simulink model "dc"  (Simulink 7.0)
settings: Solver=ode45  StartTime=0.0  StopTime=3.0  RelTol=1e-3
settings Model: Creator=User  LastModifiedBy=azad

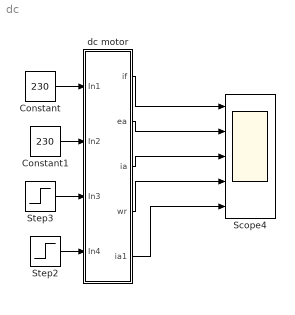
== system dc ==
  Constant : Constant  Value=230  OutDataType=sfix(16)  OutScaling=2^0
  Constant1 : Constant  Value=230  OutDataType=sfix(16)  OutScaling=2^0
  Scope4 : Scope  NumInputPorts=5
      settings: YMin=0~0~0~0~-5  YMax=1~30~400~17.5~5  SaveName=ScopeData4
  Step2 : Step  Time=1.5  After=-250  SampleTime=0
  Step3 : Step  After=250  SampleTime=0
  dc motor : Subsystem  mask{ra=0.6, rf=240, la=0.012, lf=120, laf=1.8, b=1.5, j=0.1}
      mask prompts: ra "ra(ohm)"; rf "rf(ohm)"; la "la(H)"; lf "lf(H)"; laf "laf(H)"; b "b(N.m.s)"; j "j(kg.m^2)"
  wires:
  Constant/1 -> dc motor/1(In1)
  Constant1/1 -> dc motor/2(In2)
  Step3/1 -> dc motor/3(In3)
  Step2/1 -> dc motor/4(In4)
  dc motor/1(if) -> Scope4/1
  dc motor/2(ea) -> Scope4/2
  dc motor/3(ia) -> Scope4/3
  dc motor/4(wr) -> Scope4/4
  dc motor/5(ia1) -> Scope4/5

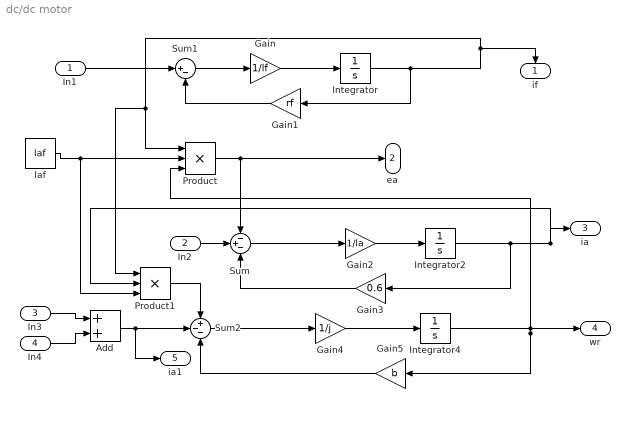
== system dc/dc motor ==
  In1 : Inport
  In2 : Inport  Port=2
  In3 : Inport  Port=3
  In4 : Inport  Port=4
  Add : Sum  OutDataType=sfix(16)  OutScaling=2^-10
  Gain : Gain  Gain=1/lf  ParameterDataType=sfix(16)  ParameterScaling=2^0  OutDataType=sfix(16)  OutScaling=2^0
  Gain1 : Gain  Orientation=left  Gain=rf  ParameterDataType=sfix(16)  ParameterScaling=2^0  OutDataType=sfix(16)  OutScaling=2^0
  Gain2 : Gain  Gain=1/la  ParameterDataType=sfix(16)  ParameterScaling=2^0  OutDataType=sfix(16)  OutScaling=2^0
  Gain3 : Gain  Orientation=left  Gain=0.6  ParameterDataType=sfix(16)  ParameterScaling=2^0  OutDataType=sfix(16)  OutScaling=2^0
  Gain4 : Gain  Gain=1/j  ParameterDataType=sfix(16)  ParameterScaling=2^0  OutDataType=sfix(16)  OutScaling=2^0
  Gain5 : Gain  Orientation=left  Gain=b  ParameterDataType=sfix(16)  ParameterScaling=2^0  OutDataType=sfix(16)  OutScaling=2^0
  Integrator : Integrator
  Integrator2 : Integrator
  Integrator4 : Integrator
  Product : Product  Inputs=3  OutDataType=sfix(16)  OutScaling=2^0  RndMeth=Zero
  Product1 : Product  Inputs=3  OutDataType=sfix(16)  OutScaling=2^0  RndMeth=Zero
  Sum : Sum  Inputs=-+-  OutDataType=sfix(16)  OutScaling=2^0
  Sum1 : Sum  Inputs=|+-  OutDataType=sfix(16)  OutScaling=2^0
  Sum2 : Sum  Inputs=+--  OutDataType=sfix(16)  OutScaling=2^0
  laf : Constant  Value=laf  OutDataType=sfix(16)  OutScaling=2^0
  if : Outport  Orientation=down
  ea : Outport  Port=2
  ia : Outport  Port=3
  wr : Outport  Port=4
  ia1 : Outport  Port=5  OutDataType=sfix(16)  OutScaling=2^0
  wires:
  Gain/1 -> Integrator/1
  Integrator/1 -> Product/1, Product1/1, if/1, Gain1/1
  Sum1/1 -> Gain/1
  Gain1/1 -> Sum1/2
  Gain2/1 -> Integrator2/1
  Sum/1 -> Gain2/1
  Integrator2/1 -> Gain3/1, Product1/2, ia/1
  Gain3/1 -> Sum/3
  Product/1 -> Sum/1, ea/1
  laf/1 -> Product/2, Product1/3
  Sum2/1 -> Gain4/1
  Gain4/1 -> Integrator4/1
  Gain5/1 -> Sum2/3
  Add/1 -> Sum2/2, ia1/1
  Product1/1 -> Sum2/1
  Integrator4/1 -> Product/3, wr/1, Gain5/1
  In1/1 -> Sum1/1
  In2/1 -> Sum/2
  In3/1 -> Add/1
  In4/1 -> Add/2
